simulink model "pstCtrl_testV2"  (R2014b)
settings: Solver=FixedStepDiscrete  SolverMode=SingleTasking  StartTime=0.0  StopTime=inf  FixedStep=0.02  RelTol=1e-3
values from neighbouring files (symbols this model uses):
  g = 9.81    [PosCntrl_Params.m]
  k_f = m*g/omega_h^2    (= 1.18520816327e-09)    [PosCntrl_Params.m]
  Kdx = 0.4    [PosCntrl_Params.m]
  Kdy = 0.4    [PosCntrl_Params.m]
  Kdz = 0.4    [PosCntrl_Params.m]
  Kpx = 1.2    [PosCntrl_Params.m]
  Kpy = 1.2    [PosCntrl_Params.m]
  Kpz = 1.2    [PosCntrl_Params.m]
  m = 0.037    [PosCntrl_Params.m]
  omega_h = 17500    [PosCntrl_Params.m]
libraries: simulink_extras x3, realtime_pacer_lib x2, simulink x1, instrumentlib x1
settings Model: CovSFcnEnable=on  Creator=rshu  LastModifiedBy=HDR
settings OptimizationCC: BlockReduction=off  BooleanDataType=off
settings DebuggingCC: SaveWithParameterizedLinksMsg=none  UnderspecifiedInitializationDetection=Classic  MergeDetectMultiDrivingBlocksExec=none  SignalResolutionControl=TryResolveAllWithWarning  SolverPrmCheckMsg=none
settings HardwareCC: TargetUnknown=on

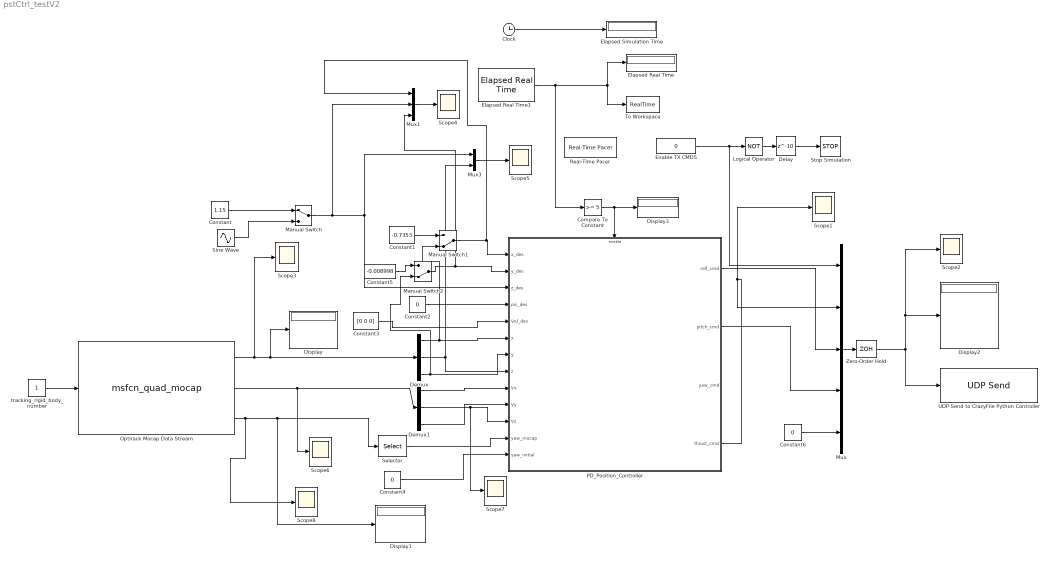
== system pstCtrl_testV2 ==
  Clock : Clock
  Compare To Constant : simulink/Logic and Bit Operations/Compare To Constant  relop=>=  const=5  OutDataTypeStr=boolean
  Constant : Constant  Value=1.15
  Constant1 : Constant  Value=-0.7353
  Constant2 : Constant  Value=0
  Constant3 : Constant  Value=[0 0 0]
  Constant4 : Constant  Value=0
  Constant5 : Constant  Value=-0.008998
  Constant6 : Constant  Value=0
  Delay : Delay  DelayLength=10  InitialCondition=0
  Demux : Demux  Outputs=3
  Demux1 : Demux  Outputs=3
  Display{,1..3} (4 alike) : Display
  Elapsed Real Time : Display
      settings: Decimation=2
  Elapsed Real Time1 : realtime_pacer_lib/Elapsed Real Time
  Elapsed Simulation Time : Display
      settings: Decimation=2
  Enable TX CMDS : Constant  Value=0
  Logical Operator : Logic  Operator=NOT  AllPortsSameDT=off  OutDataTypeStr=boolean
  Manual Switch : ManualSwitch
  Manual Switch1 : ManualSwitch  CurrentSetting=0
  Manual Switch2 : ManualSwitch  CurrentSetting=0
  Mux : Mux  Inputs=5
  Mux1 : Mux  Inputs=3
  Mux3 : Mux  Inputs=2
  Optirack Mocap Data Stream : M-S-Function  FunctionName=msfcn_quad_mocap
      mask Display:
      | image('prime41-optitrack.png');
      | color('cyan')
      | port_label('output',1,'pos (vec) [m]');
      | port_label('output',2,'vel (vec) [m/s]');
      | port_label('output',3,'orient (euler) [rad]');
      | port_label('input', 1, 'RigidBody No.')
  PD_Position_Controller : Subsystem
  Real-Time Pacer : realtime_pacer_lib/Real-Time Pacer  simTimePerRealTime=1
  Scope{1..8} (8 alike) : Scope
      Scope1 settings: YMin=60  YMax=100  SaveName=Thrust_cmd
      Scope2 settings: YMin=50468.8  YMax=55781.2  SaveName=ScopeData6
      Scope3 settings: YMin=-2  YMax=2  SaveName=Pos
      Scope4 settings: YMin=0.9  YMax=1.3  SaveName=PosDes
      Scope5 settings: YMin=1.135  YMax=1.155  SaveName=PosDes2
      Scope6 settings: YMin=-20  YMax=30  SaveName=Vel
      Scope7 settings: YMin=-20  YMax=30  SaveName=Vel1
      Scope8 settings: YMin=-20  YMax=30  SaveName=Orient
  Selector : Selector  InputPortWidth=3  Indices=[2]
  Sine Wave : Sin  Amplitude=0.2  Bias=1.3  SampleTime=0
  Stop Simulation : Stop
  To Workspace : ToWorkspace  VariableName=RealTime  SampleTime=-1
  UDP Send to CrazyFlie Python Controller : instrumentlib/UDP Send  Host=192.168.1.215  Port=51001  LocalPort=-1  EnableBlockingMode=on  ByteOrder=BigEndian
  Zero-Order Hold : ZeroOrderHold  SampleTime=0.02
  tracking_rigid_body_number : Constant
  wires:
  Optirack Mocap Data Stream/1 -> Scope3/1, Demux/1, Display/1
  Optirack Mocap Data Stream/2 -> Scope6/1, Demux1/1
  Demux/1 -> Manual Switch1/2, PD_Position_Controller/6(x)
  Demux1/1 -> PD_Position_Controller/9(Vx)
  Selector/1 -> PD_Position_Controller/12(yaw_mocap)
  Constant2/1 -> PD_Position_Controller/4(psi_des)
  Constant3/1 -> PD_Position_Controller/5(Vel_des)
  Constant4/1 -> PD_Position_Controller/13(yaw_initial)
  Mux/1 -> Zero-Order Hold/1
  Demux/2 -> Mux3/2, PD_Position_Controller/8(z)
  Demux/3 -> PD_Position_Controller/7(y), Manual Switch2/2
  Demux1/3 -> PD_Position_Controller/10(Vy)
  Manual Switch/1 -> Mux1/2, PD_Position_Controller/3(z_des), Mux3/1
  Optirack Mocap Data Stream/3 -> Scope8/1, Display1/1, Selector/1
  Clock/1 -> Elapsed Simulation Time/1
  Elapsed Real Time1/1 -> To Workspace/1, Elapsed Real Time/1, Compare To Constant/1
  PD_Position_Controller/4(thrust_cmd) -> Scope1/1, Mux/2
  tracking_rigid_body_number/1 -> Optirack Mocap Data Stream/1
  Zero-Order Hold/1 -> UDP Send to CrazyFlie Python Controller/1, Scope2/1, Display2/1
  Enable TX CMDS/1 -> Mux/1, Logical Operator/1
  Mux3/1 -> Scope5/1
  Logical Operator/1 -> Delay/1
  Delay/1 -> Stop Simulation/1
  Constant/1 -> Manual Switch/1
  Sine Wave/1 -> Manual Switch/2
  Compare To Constant/1 -> Display3/1, PD_Position_Controller/Enable
  Demux1/2 -> Scope7/1, PD_Position_Controller/11(Vz)
  Mux1/1 -> Scope4/1
  Manual Switch1/1 -> Mux1/1, PD_Position_Controller/1(x_des)
  Constant1/1 -> Manual Switch1/1
  Constant5/1 -> Manual Switch2/1
  Manual Switch2/1 -> PD_Position_Controller/2(y_des), Mux1/3
  PD_Position_Controller/2(pitch_cmd) -> Mux/4
  PD_Position_Controller/1(roll_cmd) -> Mux/3
  Constant6/1 -> Mux/5

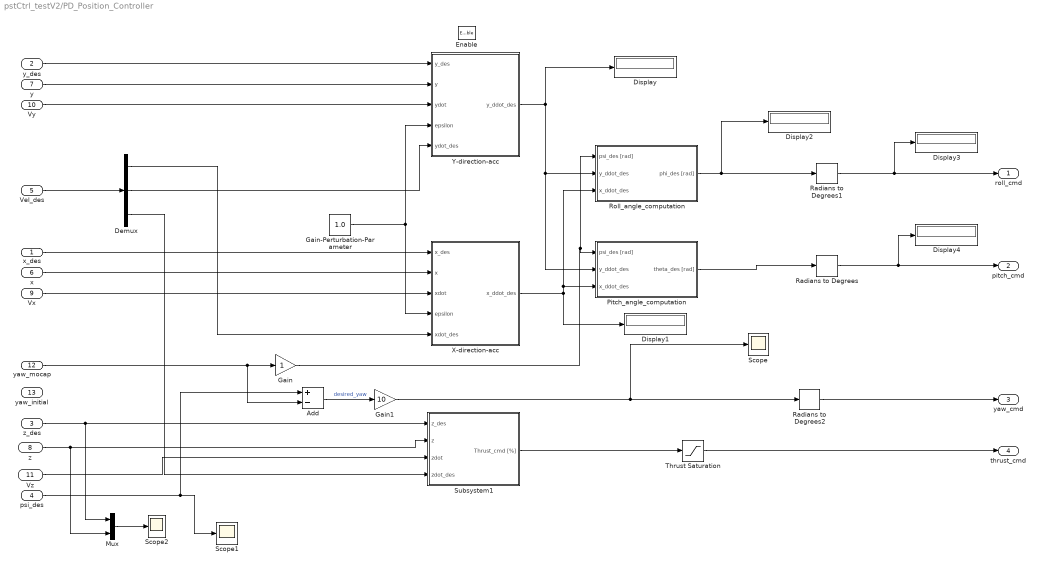
== system pstCtrl_testV2/PD_Position_Controller ==
  x_des : Inport
  y_des : Inport  Port=2
  z_des : Inport  Port=3
  psi_des : Inport  Port=4
  Vel_des : Inport  Port=5
  x : Inport  Port=6
  y : Inport  Port=7
  z : Inport  Port=8
  Vx : Inport  Port=9
  Vy : Inport  Port=10
  Vz : Inport  Port=11
  yaw_mocap : Inport  Port=12
  yaw_initial : Inport  Port=13
  Enable : EnablePort
  Add : Sum  Inputs=+-
  Demux : Demux  Outputs=3
  Display{,1..4} (5 alike) : Display
  Gain : Gain
  Gain-Perturbation-Parameter : Constant  Value=1.0
  Gain1 : Gain  Gain=10
  Mux : Mux  Inputs=2
  Pitch_angle_computation : Subsystem
  Radians to Degrees : simulink_extras/Transformations/Radians to Degrees
  Radians to Degrees1 : simulink_extras/Transformations/Radians to Degrees
  Radians to Degrees2 : simulink_extras/Transformations/Radians to Degrees
  Roll_angle_computation : Subsystem
  Scope : Scope
      settings: YMin=-1  YMax=1.5  SaveName=ScopeData35
  Scope1 : Scope
      settings: SaveName=ScopeData37
  Scope2 : Scope
      settings: YMin=0.65  YMax=1  SaveName=ScopeData5
  Subsystem1 : Subsystem
  Thrust Saturation : Saturate  UpperLimit=100  LowerLimit=0
  X-direction-acc : Subsystem
  Y-direction-acc : Subsystem
  roll_cmd : Outport  InitialOutput=0
  pitch_cmd : Outport  Port=2  InitialOutput=0
  yaw_cmd : Outport  Port=3  InitialOutput=0
  thrust_cmd : Outport  Port=4  InitialOutput=50
  wires:
  Gain-Perturbation-Parameter/1 -> X-direction-acc/4("epsilon "), Y-direction-acc/4("epsilon ")
  X-direction-acc/1(x_ddot_des) -> Display1/1, Roll_angle_computation/3("x_ddot_des "), Pitch_angle_computation/3("x_ddot_des ")
  Y-direction-acc/1(y_ddot_des) -> Pitch_angle_computation/2(y_ddot_des), Roll_angle_computation/2(y_ddot_des), Display/1
  Vz/1 -> Subsystem1/3("zdot ")
  y/1 -> Y-direction-acc/2(y)
  Vx/1 -> X-direction-acc/3("xdot ")
  x/1 -> X-direction-acc/2(x)
  Add/1 -> Gain1/1  "desired_yaw"
  psi_des/1 -> Add/1, Scope1/1
  z_des/1 -> Mux/1, Subsystem1/1(z_des)
  yaw_mocap/1 -> Add/2, Gain/1
  Gain/1 -> Pitch_angle_computation/1("psi_des [rad] "), Roll_angle_computation/1("psi_des [rad] ")
  x_des/1 -> X-direction-acc/1(x_des)
  y_des/1 -> Y-direction-acc/1(y_des)
  Vel_des/1 -> Demux/1
  Demux/1 -> X-direction-acc/5(xdot_des)
  Demux/3 -> Subsystem1/4(zdot_des)
  Roll_angle_computation/1("phi_des [rad] ") -> Radians to Degrees1/1, Display2/1
  Pitch_angle_computation/1("theta_des [rad] ") -> Radians to Degrees/1
  Mux/1 -> Scope2/1
  z/1 -> Mux/2, Subsystem1/2(z)
  Subsystem1/1(Thrust_cmd [%]) -> Thrust Saturation/1
  Thrust Saturation/1 -> thrust_cmd/1
  Vy/1 -> Y-direction-acc/3("ydot ")
  Demux/2 -> Y-direction-acc/5(ydot_des)
  Radians to Degrees/1 -> Display4/1, pitch_cmd/1
  Radians to Degrees1/1 -> Display3/1, roll_cmd/1
  Radians to Degrees2/1 -> yaw_cmd/1
  Gain1/1 -> Radians to Degrees2/1, Scope/1

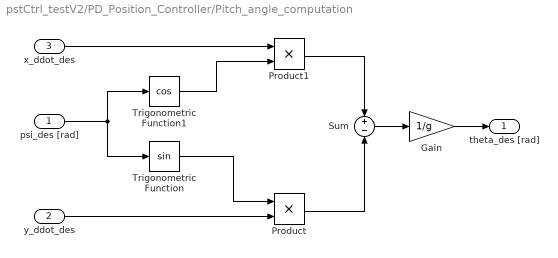
== system pstCtrl_testV2/PD_Position_Controller/Pitch_angle_computation ==
  "psi_des [rad] " : Inport
  y_ddot_des : Inport  Port=2
  "x_ddot_des " : Inport  Port=3
  Gain : Gain  Gain=1/g
  Product : Product
  Product1 : Product
  Sum : Sum  Inputs=+-
  Trigonometric Function : Trigonometry
  Trigonometric Function1 : Trigonometry  Operator=cos
  "theta_des [rad] " : Outport
  wires:
  "psi_des [rad] "/1 -> Trigonometric Function1/1, Trigonometric Function/1
  y_ddot_des/1 -> Product/2
  Trigonometric Function/1 -> Product/1
  "x_ddot_des "/1 -> Product1/1
  Trigonometric Function1/1 -> Product1/2
  Product1/1 -> Sum/1
  Product/1 -> Sum/2
  Sum/1 -> Gain/1
  Gain/1 -> "theta_des [rad] "/1

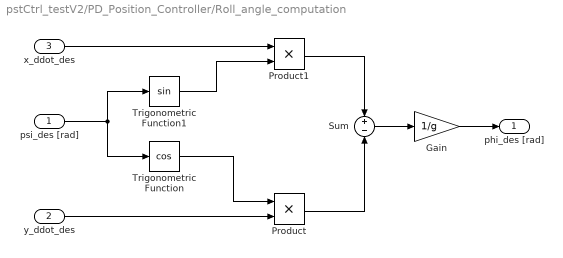
== system pstCtrl_testV2/PD_Position_Controller/Roll_angle_computation ==
  "psi_des [rad] " : Inport
  y_ddot_des : Inport  Port=2
  "x_ddot_des " : Inport  Port=3
  Gain : Gain  Gain=1/g
  Product : Product
  Product1 : Product
  Sum : Sum  Inputs=+-
  Trigonometric Function : Trigonometry  Operator=cos
  Trigonometric Function1 : Trigonometry
  "phi_des [rad] " : Outport
  wires:
  "psi_des [rad] "/1 -> Trigonometric Function1/1, Trigonometric Function/1
  y_ddot_des/1 -> Product/2
  Trigonometric Function/1 -> Product/1
  "x_ddot_des "/1 -> Product1/1
  Trigonometric Function1/1 -> Product1/2
  Product1/1 -> Sum/1
  Product/1 -> Sum/2
  Sum/1 -> Gain/1
  Gain/1 -> "phi_des [rad] "/1

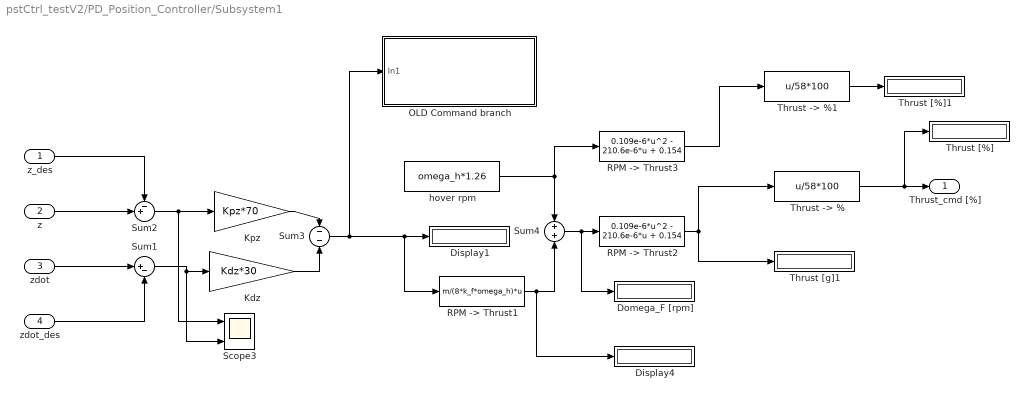
== system pstCtrl_testV2/PD_Position_Controller/Subsystem1 ==
  z_des : Inport
  z : Inport  Port=2
  "zdot " : Inport  Port=3
  zdot_des : Inport  Port=4
  Display1 : Display
  Display4 : Display
  Domega_F [rpm] : Display
  Kdz : Gain  Gain=Kdz*30
  Kpz : Gain  Gain=Kpz*70
  OLD Command branch : Subsystem
  "RPM -> Thrust1" : Fcn  Expr=m/(8*k_f*omega_h)*u
  "RPM -> Thrust2" : Fcn  Expr=0.109e-6*u^2 - 210.6e-6*u + 0.154
  "RPM -> Thrust3" : Fcn  Expr=0.109e-6*u^2 - 210.6e-6*u + 0.154
  Scope3 : Scope  NumInputPorts=2
      settings: YMin=-0.1~0.2855  YMax=0.4~0.289  SaveName=ScopeData7
  Sum1 : Sum  Inputs=|+-
  Sum2 : Sum  Inputs=-+|
  Sum3 : Sum  Inputs=--
  Sum4 : Sum  Inputs=+|+
  Thrust [%] : Display
  Thrust [%]1 : Display
  Thrust [g]1 : Display
  "Thrust -> %" : Fcn  Expr=u/58*100
  "Thrust -> %1" : Fcn  Expr=u/58*100
  hover rpm : Constant  Value=omega_h*1.26
  Thrust_cmd [%] : Outport
  wires:
  "zdot "/1 -> Sum1/1
  zdot_des/1 -> Sum1/2
  Sum1/1 -> Scope3/2, Kdz/1
  z/1 -> Sum2/2
  z_des/1 -> Sum2/1
  Sum2/1 -> Scope3/1, Kpz/1
  Kpz/1 -> Sum3/1
  Kdz/1 -> Sum3/2
  Sum3/1 -> OLD Command branch/1(In1), "RPM -> Thrust1"/1, Display1/1
  "Thrust -> %"/1 -> Thrust [%]/1, Thrust_cmd [%]/1
  "RPM -> Thrust1"/1 -> Display4/1, Sum4/2
  "RPM -> Thrust2"/1 -> "Thrust -> %"/1, Thrust [g]1/1
  Sum4/1 -> Domega_F [rpm]/1, "RPM -> Thrust2"/1
  hover rpm/1 -> Sum4/1, "RPM -> Thrust3"/1
  "RPM -> Thrust3"/1 -> "Thrust -> %1"/1
  "Thrust -> %1"/1 -> Thrust [%]1/1

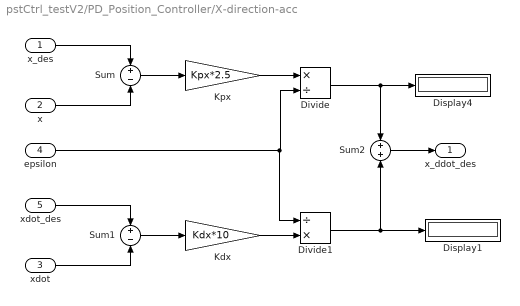
== system pstCtrl_testV2/PD_Position_Controller/X-direction-acc ==
  x_des : Inport
  x : Inport  Port=2
  "xdot " : Inport  Port=3
  "epsilon " : Inport  Port=4
  xdot_des : Inport  Port=5
  Display1 : Display
  Display4 : Display
  Divide : Product  Inputs=*/
  Divide1 : Product  Inputs=/*
  Kdx : Gain  Gain=Kdx*10
  Kpx : Gain  Gain=Kpx*2.5
  Sum : Sum  Inputs=+-
  Sum1 : Sum  Inputs=+-
  Sum2 : Sum
  x_ddot_des : Outport
  wires:
  x_des/1 -> Sum/1
  x/1 -> Sum/2
  Sum/1 -> Kpx/1
  Kpx/1 -> Divide/1
  "epsilon "/1 -> Divide1/1, Divide/2
  xdot_des/1 -> Sum1/1
  "xdot "/1 -> Sum1/2
  Sum1/1 -> Kdx/1
  Kdx/1 -> Divide1/2
  Divide/1 -> Display4/1, Sum2/1
  Divide1/1 -> Display1/1, Sum2/2
  Sum2/1 -> x_ddot_des/1

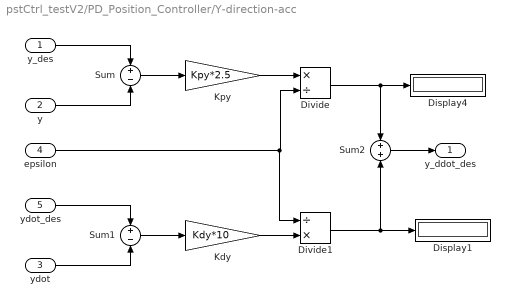
== system pstCtrl_testV2/PD_Position_Controller/Y-direction-acc ==
  y_des : Inport
  y : Inport  Port=2
  "ydot " : Inport  Port=3
  "epsilon " : Inport  Port=4
  ydot_des : Inport  Port=5
  Display1 : Display
  Display4 : Display
  Divide : Product  Inputs=*/
  Divide1 : Product  Inputs=/*
  Kdy : Gain  Gain=Kdy*10
  Kpy : Gain  Gain=Kpy*2.5
  Sum : Sum  Inputs=+-
  Sum1 : Sum  Inputs=+-
  Sum2 : Sum
  y_ddot_des : Outport
  wires:
  y_des/1 -> Sum/1
  y/1 -> Sum/2
  Sum/1 -> Kpy/1
  Kpy/1 -> Divide/1
  "epsilon "/1 -> Divide1/1, Divide/2
  ydot_des/1 -> Sum1/1
  "ydot "/1 -> Sum1/2
  Sum1/1 -> Kdy/1
  Kdy/1 -> Divide1/2
  Divide/1 -> Display4/1, Sum2/1
  Divide1/1 -> Display1/1, Sum2/2
  Sum2/1 -> y_ddot_des/1

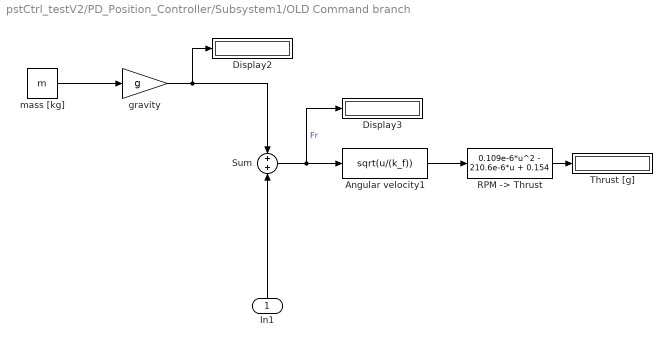
== system pstCtrl_testV2/PD_Position_Controller/Subsystem1/OLD Command branch ==
  In1 : Inport
  Angular velocity1 : Fcn  Expr=sqrt(u/(k_f))
  Display2 : Display
  Display3 : Display
  "RPM -> Thrust" : Fcn  Expr=0.109e-6*u^2 - 210.6e-6*u + 0.154
  Sum : Sum  Inputs=+|+
  Thrust [g] : Display
  gravity : Gain  Gain=g
  "mass [kg] " : Constant  Value=m
  wires:
  In1/1 -> Sum/2
  "mass [kg] "/1 -> gravity/1
  Sum/1 -> Display3/1, Angular velocity1/1  "Fr"
  gravity/1 -> Display2/1, Sum/1
  Angular velocity1/1 -> "RPM -> Thrust"/1
  "RPM -> Thrust"/1 -> Thrust [g]/1
